simulink model "gm_flightController"  (R2018b)
settings: Solver=ode3  StartTime=0  StopTime=TFinal  FixedStep=Ts  RelTol=1e-3  EnableMultiTasking=on
libraries: hdlmdlgenlib x14
(part 1 of 2)
settings Model: Creator=The MathWorks, Inc.  LastModifiedBy=asus
settings SolverCC: MinimalZcImpactIntegration=on
settings DataIOCC: LimitDataPoints=on  SaveFormat=Array
settings OptimizationCC: BlockReduction=off  ConditionallyExecuteInputs=off  DefaultParameterBehavior=Inlined  BufferReuse=off  PassReuseOutputArgsThreshold=0
settings DebuggingCC: AlgebraicLoopMsg=none  InheritedTsInSrcMsg=none  ParameterPrecisionLossMsg=none  ParameterTunabilityLossMsg=error  UnconnectedInputMsg=none  UnconnectedOutputMsg=none  UnconnectedLineMsg=none  BusObjectLabelMismatch=error  LibraryContextMissingDiagnostic=none  SFUnexpectedBacktrackingDiag=warning  SFNoUnconditionalDefaultTransitionDiag=warning  SFExecutionAtInitializationDiag=none
settings HardwareCC: ProdBitPerPointer=32  ProdBitPerSizeT=32  ProdBitPerPtrDiffT=32  ProdLargestAtomicInteger=Long  ProdWordSize=32  ProdHWDeviceType=ARM Compatible->ARM 9
settings ModelReferenceCC: ModelReferenceNumInstancesAllowed=Single  PropagateSignalLabelsOutOfModel=off
settings SFSimCC: SimUseLocalCustomCode=off
settings RTWCC: Description=Generic Real-Time Target  GenerateReport=on  RTWUseLocalCustomCode=off  LaunchReport=on
settings CodeAppCC: ForceParamTrailComments=on  MaxIdLength=63  OperatorAnnotations=on  StateflowObjectComments=on  MATLABSourceComments=on
settings GRTTargetCC: TargetLangStandard=C89/C90 (ANSI)
settings ConfigComp: CovMetricSettings=dw  CovHtmlReporting=on  CovSaveCumulativeToWorkspaceVar=on  CovSaveSingleToWorkspaceVar=on  CovExternalEMLEnable=off  CovSFcnEnable=off

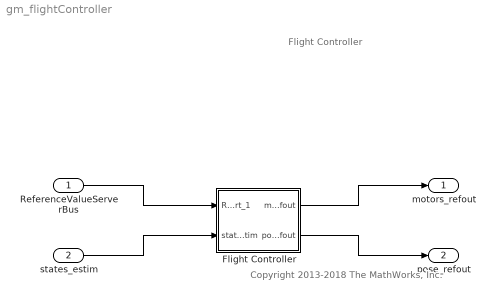
== system gm_flightController ==
  note: Copyright 2013-2018 The MathWorks, Inc.
  note: Flight Controller
  ReferenceValueServerBus : Inport  OutDataTypeStr=Bus: CommandBus  SampleTime=0.005  BusOutputAsStruct=on
  states_estim : Inport  Port=2  OutDataTypeStr=Bus: statesEstim_t  SampleTime=0.005  BusOutputAsStruct=on
  Flight Controller : Subsystem
  motors_refout : Outport
  pose_refout : Outport  Port=2
  wires:
  ReferenceValueServerBus/1 -> Flight Controller/1(ReferenceValueServerBus_Inport_1)
  states_estim/1 -> Flight Controller/2(states_estim)
  Flight Controller/1(motors_refout) -> motors_refout/1
  Flight Controller/2(pose_refout) -> pose_refout/1

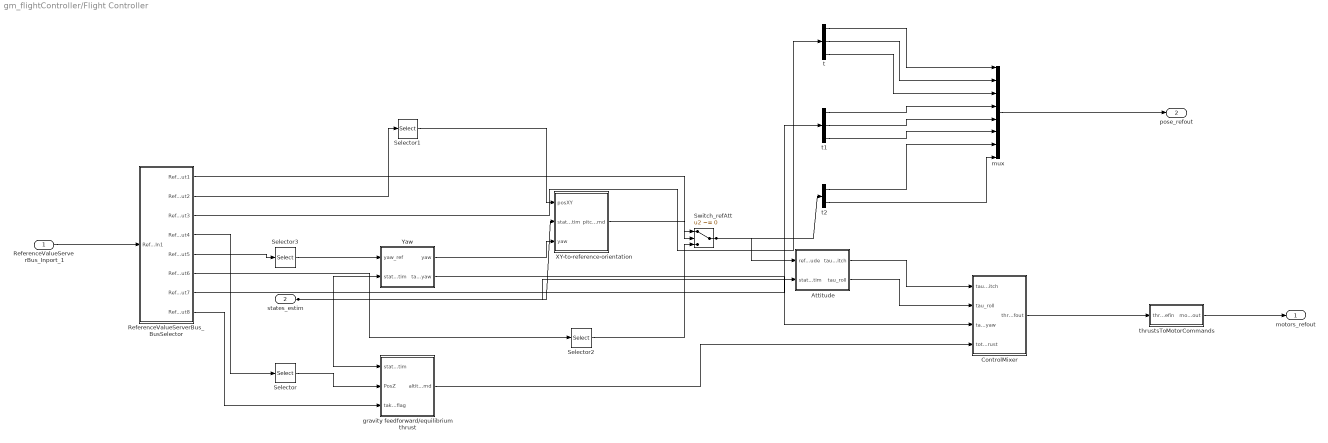
== system gm_flightController/Flight Controller ==
  ReferenceValueServerBus_Inport_1 : Inport  SampleTime=0.005
  states_estim : Inport  Port=2  SampleTime=0.005
  Attitude : Subsystem
  ControlMixer : Subsystem
  ReferenceValueServerBus_BusSelector : Subsystem
  Selector : Selector  SampleTime=0.005  IndexOptions=Index vector (dialog)  Indices=double(3)  OutputSizes=double(1)
  Selector1 : Selector  SampleTime=0.005  IndexOptions=Index vector (dialog)  Indices=double([1 2])  OutputSizes=double(1)
  Selector2 : Selector  SampleTime=0.005  IndexOptions=Index vector (dialog)  Indices=double([2 3])  OutputSizes=double(1)
  Selector3 : Selector  SampleTime=0.005  IndexOptions=Index vector (dialog)  Indices=double(1)  OutputSizes=double(1)
  Switch_refAtt : Switch  Criteria=u2 ~= 0  Threshold=double(0)  OutDataTypeStr=single  SampleTime=0.005
  XY-to-reference-orientation : Subsystem
  Yaw : Subsystem
  gravity feedforward/equilibrium thrust : Subsystem
  mux : Mux  Inputs=8
  t : Demux  Outputs=3
  t1 : Demux  Outputs=3
  t2 : Demux  Outputs=2
  thrustsToMotorCommands : Subsystem
  motors_refout : Outport
  pose_refout : Outport  Port=2
  wires:
  ReferenceValueServerBus_Inport_1/1 -> ReferenceValueServerBus_BusSelector/1(ReferenceValueServerBus_BusSelector_In1)
  states_estim/1 -> gravity feedforward/equilibrium thrust/1(states_estim), Attitude/2(states_estim), XY-to-reference-orientation/2(states_estim), Yaw/2(states_estim)
  Attitude/1(tau_pitch) -> ControlMixer/1(tau_pitch)
  Attitude/2(tau_roll) -> ControlMixer/2(tau_roll)
  ControlMixer/1(thrusts_refout) -> thrustsToMotorCommands/1(thrusts_refin)
  mux/1 -> pose_refout/1
  ReferenceValueServerBus_BusSelector/1(ReferenceValueServerBus_BusSelector_Out1) -> Switch_refAtt/2
  ReferenceValueServerBus_BusSelector/2(ReferenceValueServerBus_BusSelector_Out2) -> Selector1/1
  ReferenceValueServerBus_BusSelector/3(ReferenceValueServerBus_BusSelector_Out3) -> t/1
  ReferenceValueServerBus_BusSelector/4(ReferenceValueServerBus_BusSelector_Out4) -> Selector/1
  ReferenceValueServerBus_BusSelector/5(ReferenceValueServerBus_BusSelector_Out5) -> Selector3/1
  ReferenceValueServerBus_BusSelector/6(ReferenceValueServerBus_BusSelector_Out6) -> Selector2/1
  ReferenceValueServerBus_BusSelector/7(ReferenceValueServerBus_BusSelector_Out7) -> t1/1
  ReferenceValueServerBus_BusSelector/8(ReferenceValueServerBus_BusSelector_Out8) -> gravity feedforward/equilibrium thrust/3(takeoff_flag)
  Selector/1 -> gravity feedforward/equilibrium thrust/2(PosZ)
  Selector1/1 -> XY-to-reference-orientation/1(posXY)
  Selector2/1 -> Switch_refAtt/3
  Selector3/1 -> Yaw/1(yaw_ref)
  Switch_refAtt/1 -> t2/1, Attitude/1(refAttitude)
  XY-to-reference-orientation/1(pitch_roll_cmd) -> Switch_refAtt/1
  Yaw/1(yaw) -> XY-to-reference-orientation/3(yaw)
  Yaw/2(tau_yaw) -> ControlMixer/3(tau_yaw)
  gravity feedforward/equilibrium thrust/1(altitude_cmd) -> ControlMixer/4(totalThrust)
  thrustsToMotorCommands/1(motors_cmdout) -> motors_refout/1
  t/1 -> mux/1
  t/2 -> mux/2
  t/3 -> mux/3
  t1/1 -> mux/4
  t1/2 -> mux/5
  t1/3 -> mux/6
  t2/1 -> mux/7
  t2/2 -> mux/8

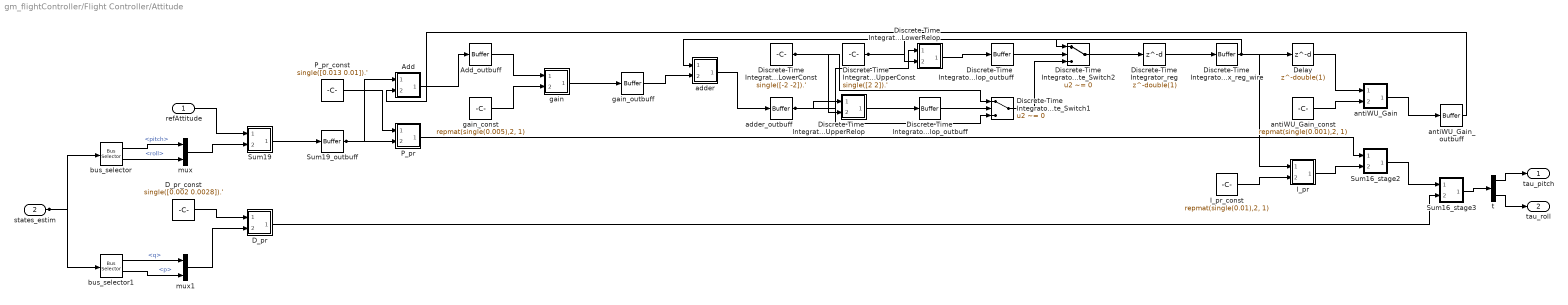
== system gm_flightController/Flight Controller/Attitude ==
  refAttitude : Inport  OutDataTypeStr=single  PortDimensions=[2]  SampleTime=0.005
  states_estim : Inport  Port=2  SampleTime=0.005
  Add : Subsystem
      mask Display: disp('NFP\nadd');
  Add_outbuff : hdlmdlgenlib/Buffer
      settings: SourceProductName=HDL Coder  SourceProductBaseCode=HD
  D_pr : Subsystem
      mask Display: disp('NFP\nmul');
  D_pr_const : Constant  Value=single([0.002 0.0028]).'  OutDataTypeStr=single  SampleTime=-1
  Delay : Delay  DelayLength=double(1)  InitialCondition=0  InputProcessing=Inherited  SampleTime=0.005
  Discrete-Time Integrator_reg : Delay  DelayLength=double(1)  InitialCondition=0  InputProcessing=Inherited  SampleTime=0.005
  Discrete-Time Integrator_saturate_LowerConst : Constant  Value=single([-2 -2]).'  OutDataTypeStr=single  SampleTime=-1
  Discrete-Time Integrator_saturate_LowerRelop : Subsystem
      mask Display: disp('NFP\nrelop');
  Discrete-Time Integrator_saturate_LowerRelop_outbuff : hdlmdlgenlib/Buffer
      settings: SourceProductName=HDL Coder  SourceProductBaseCode=HD
  Discrete-Time Integrator_saturate_Switch1 : Switch  Criteria=u2 ~= 0  Threshold=double(0)  OutDataTypeStr=single  SampleTime=0.005
  Discrete-Time Integrator_saturate_Switch2 : Switch  Criteria=u2 ~= 0  Threshold=double(0)  OutDataTypeStr=single  SampleTime=0.005
  Discrete-Time Integrator_saturate_UpperConst : Constant  Value=single([2 2]).'  OutDataTypeStr=single  SampleTime=-1
  Discrete-Time Integrator_saturate_UpperRelop : Subsystem
      mask Display: disp('NFP\nrelop');
  Discrete-Time Integrator_saturate_UpperRelop_outbuff : hdlmdlgenlib/Buffer
      settings: SourceProductName=HDL Coder  SourceProductBaseCode=HD
  Discrete-Time Integrator_x_reg_wire : hdlmdlgenlib/Buffer
      settings: SourceProductName=HDL Coder  SourceProductBaseCode=HD
  I_pr : Subsystem
      mask Display: disp('NFP\nmul');
  I_pr_const : Constant  Value=repmat(single(0.01),2, 1)  OutDataTypeStr=single  SampleTime=-1
  P_pr : Subsystem
      mask Display: disp('NFP\nmul');
  P_pr_const : Constant  Value=single([0.013 0.01]).'  OutDataTypeStr=single  SampleTime=-1
  Sum16_stage2 : Subsystem
      mask Display: disp('NFP\nadd');
  Sum16_stage3 : Subsystem
      mask Display: disp('NFP\nadd');
  Sum19 : Subsystem
      mask Display: disp('NFP\nadd');
  Sum19_outbuff : hdlmdlgenlib/Buffer
      settings: SourceProductName=HDL Coder  SourceProductBaseCode=HD
  adder : Subsystem
      mask Display: disp('NFP\nadd');
  adder_outbuff : hdlmdlgenlib/Buffer
      settings: SourceProductName=HDL Coder  SourceProductBaseCode=HD
  antiWU_Gain : Subsystem
      mask Display: disp('NFP\nmul');
  antiWU_Gain_const : Constant  Value=repmat(single(0.001),2, 1)  OutDataTypeStr=single  SampleTime=-1
  antiWU_Gain_outbuff : hdlmdlgenlib/Buffer
      settings: SourceProductName=HDL Coder  SourceProductBaseCode=HD
  bus_selector : BusSelector  OutputSignals=pitch,roll
  bus_selector1 : BusSelector  OutputSignals=q,p
  gain : Subsystem
      mask Display: disp('NFP\nmul');
  gain_const : Constant  Value=repmat(single(0.005),2, 1)  OutDataTypeStr=single  SampleTime=-1
  gain_outbuff : hdlmdlgenlib/Buffer
      settings: SourceProductName=HDL Coder  SourceProductBaseCode=HD
  mux : Mux  Inputs=2
  mux1 : Mux  Inputs=2
  t : Demux  Outputs=2
  tau_pitch : Outport
  tau_roll : Outport  Port=2
  wires:
  refAttitude/1 -> Sum19/1(In1)
  states_estim/1 -> bus_selector1/1, bus_selector/1
  Add_outbuff/1 -> gain/1(In1)
  bus_selector/1 -> mux/1  "<pitch>"
  bus_selector/2 -> mux/2  "<roll>"
  bus_selector1/1 -> mux1/1  "<q>"
  bus_selector1/2 -> mux1/2  "<p>"
  Delay/1 -> antiWU_Gain/1(In1)
  Discrete-Time Integrator_x_reg_wire/1 -> I_pr/1(In1), adder/1(In1), Delay/1
  mux/1 -> Sum19/2(In2)
  mux1/1 -> D_pr/2(In2)
  Sum19_outbuff/1 -> P_pr/2(In2), Add/1(In1)
  antiWU_Gain_outbuff/1 -> Add/2(In2)
  gain_outbuff/1 -> adder/2(In2)
  adder_outbuff/1 -> Discrete-Time Integrator_saturate_LowerRelop/1(In1), Discrete-Time Integrator_saturate_UpperRelop/1(In1), Discrete-Time Integrator_saturate_Switch1/3
  Discrete-Time Integrator_saturate_Switch2/1 -> Discrete-Time Integrator_reg/1
  Discrete-Time Integrator_saturate_LowerConst/1 -> Discrete-Time Integrator_saturate_UpperRelop/2(In2), Discrete-Time Integrator_saturate_Switch1/1
  Discrete-Time Integrator_saturate_UpperConst/1 -> Discrete-Time Integrator_saturate_LowerRelop/2(In2), Discrete-Time Integrator_saturate_Switch2/1
  Discrete-Time Integrator_saturate_UpperRelop_outbuff/1 -> Discrete-Time Integrator_saturate_Switch1/2
  Discrete-Time Integrator_saturate_LowerRelop_outbuff/1 -> Discrete-Time Integrator_saturate_Switch2/2
  Discrete-Time Integrator_saturate_Switch1/1 -> Discrete-Time Integrator_saturate_Switch2/3
  Discrete-Time Integrator_reg/1 -> Discrete-Time Integrator_x_reg_wire/1
  t/1 -> tau_pitch/1
  t/2 -> tau_roll/1
  D_pr_const/1 -> D_pr/1(In1)
  gain_const/1 -> gain/2(In2)
  I_pr_const/1 -> I_pr/2(In2)
  P_pr_const/1 -> P_pr/1(In1)
  antiWU_Gain_const/1 -> antiWU_Gain/2(In2)
  adder/1(Out1) -> adder_outbuff/1
  Discrete-Time Integrator_saturate_UpperRelop/1(Out1) -> Discrete-Time Integrator_saturate_UpperRelop_outbuff/1
  Discrete-Time Integrator_saturate_LowerRelop/1(Out1) -> Discrete-Time Integrator_saturate_LowerRelop_outbuff/1
  Add/1(Out1) -> Add_outbuff/1
  Sum16_stage2/1(Out1) -> Sum16_stage3/1(In1)
  Sum16_stage3/1(Out1) -> t/1
  Sum19/1(Out1) -> Sum19_outbuff/1
  D_pr/1(Out1) -> Sum16_stage3/2(In2)
  gain/1(Out1) -> gain_outbuff/1
  I_pr/1(Out1) -> Sum16_stage2/2(In2)
  P_pr/1(Out1) -> Sum16_stage2/1(In1)
  antiWU_Gain/1(Out1) -> antiWU_Gain_outbuff/1

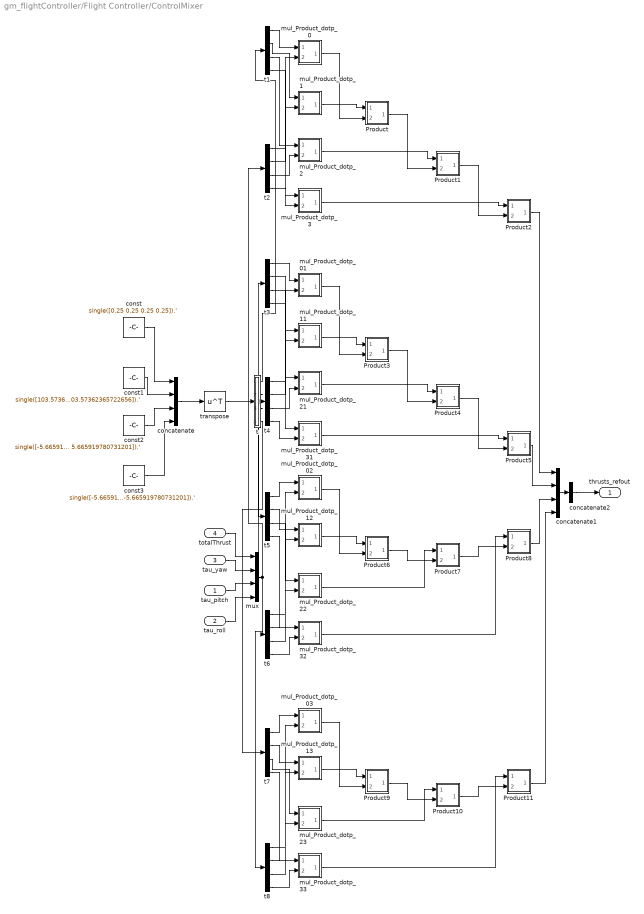
== system gm_flightController/Flight Controller/ControlMixer ==
  tau_pitch : Inport  OutDataTypeStr=single  PortDimensions=1  SampleTime=0.005
  tau_roll : Inport  Port=2  OutDataTypeStr=single  PortDimensions=1  SampleTime=0.005
  tau_yaw : Inport  Port=3  OutDataTypeStr=single  PortDimensions=1  SampleTime=0.005
  totalThrust : Inport  Port=4  OutDataTypeStr=single  PortDimensions=1  SampleTime=0.005
  Product : Subsystem
      mask Display: disp('NFP\nadd');
  Product1 : Subsystem
      mask Display: disp('NFP\nadd');
  Product10 : Subsystem
      mask Display: disp('NFP\nadd');
  Product11 : Subsystem
      mask Display: disp('NFP\nadd');
  Product2 : Subsystem
      mask Display: disp('NFP\nadd');
  Product3 : Subsystem
      mask Display: disp('NFP\nadd');
  Product4 : Subsystem
      mask Display: disp('NFP\nadd');
  Product5 : Subsystem
      mask Display: disp('NFP\nadd');
  Product6 : Subsystem
      mask Display: disp('NFP\nadd');
  Product7 : Subsystem
      mask Display: disp('NFP\nadd');
  Product8 : Subsystem
      mask Display: disp('NFP\nadd');
  Product9 : Subsystem
      mask Display: disp('NFP\nadd');
  concatenate : Concatenate  NumInputs=4  Mode=Multidimensional array  ConcatenateDimension=2
  concatenate1 : Concatenate  NumInputs=4
  concatenate2 : Concatenate  NumInputs=1  Mode=Multidimensional array  ConcatenateDimension=2
  const : Constant  Value=single([0.25 0.25 0.25 0.25]).'  OutDataTypeStr=single  SampleTime=-1
  const1 : Constant  Value=single([103.57362365722656 -103.57362365722656 103.57362365722656 -103.57362365722656]).'  OutDataTypeStr=single  SampleTime=-1
  const2 : Constant  Value=single([-5.665919780731201 -5.665919780731201 5.665919780731201 5.665919780731201]).'  OutDataTypeStr=single  SampleTime=-1
  const3 : Constant  Value=single([-5.665919780731201 5.665919780731201 5.665919780731201 -5.665919780731201]).'  OutDataTypeStr=single  SampleTime=-1
  mul_Product_dotp_0 : Subsystem
      mask Display: disp('NFP\nmul');
  mul_Product_dotp_01 : Subsystem
      mask Display: disp('NFP\nmul');
  mul_Product_dotp_02 : Subsystem
      mask Display: disp('NFP\nmul');
  mul_Product_dotp_03 : Subsystem
      mask Display: disp('NFP\nmul');
  mul_Product_dotp_1 : Subsystem
      mask Display: disp('NFP\nmul');
  mul_Product_dotp_11 : Subsystem
      mask Display: disp('NFP\nmul');
  mul_Product_dotp_12 : Subsystem
      mask Display: disp('NFP\nmul');
  mul_Product_dotp_13 : Subsystem
      mask Display: disp('NFP\nmul');
  mul_Product_dotp_2 : Subsystem
      mask Display: disp('NFP\nmul');
  mul_Product_dotp_21 : Subsystem
      mask Display: disp('NFP\nmul');
  mul_Product_dotp_22 : Subsystem
      mask Display: disp('NFP\nmul');
  mul_Product_dotp_23 : Subsystem
      mask Display: disp('NFP\nmul');
  mul_Product_dotp_3 : Subsystem
      mask Display: disp('NFP\nmul');
  mul_Product_dotp_31 : Subsystem
      mask Display: disp('NFP\nmul');
  mul_Product_dotp_32 : Subsystem
      mask Display: disp('NFP\nmul');
  mul_Product_dotp_33 : Subsystem
      mask Display: disp('NFP\nmul');
  mux : Mux
  t : Subsystem
  t{1..8} (8 alike) : Demux
  transpose : Math  Operator=transpose  SaturateOnIntegerOverflow=on
  thrusts_refout : Outport
  wires:
  tau_pitch/1 -> mux/3
  tau_roll/1 -> mux/4
  tau_yaw/1 -> mux/2
  totalThrust/1 -> mux/1
  mux/1 -> t8/1, t6/1, t4/1, t2/1
  concatenate2/1 -> thrusts_refout/1
  concatenate/1 -> transpose/1
  const/1 -> concatenate/1
  const1/1 -> concatenate/2
  const2/1 -> concatenate/3
  const3/1 -> concatenate/4
  transpose/1 -> t/1(in0)
  t/1(out0) -> t1/1
  t/2(out1) -> t3/1
  t/3(out2) -> t5/1
  t/4(out3) -> t7/1
  t1/1 -> mul_Product_dotp_0/1(In1)
  t1/2 -> mul_Product_dotp_1/1(In1)
  t1/3 -> mul_Product_dotp_2/1(In1)
  t1/4 -> mul_Product_dotp_3/1(In1)
  t2/1 -> mul_Product_dotp_0/2(In2)
  t2/2 -> mul_Product_dotp_1/2(In2)
  t2/3 -> mul_Product_dotp_2/2(In2)
  t2/4 -> mul_Product_dotp_3/2(In2)
  t3/1 -> mul_Product_dotp_01/1(In1)
  t3/2 -> mul_Product_dotp_11/1(In1)
  t3/3 -> mul_Product_dotp_21/1(In1)
  t3/4 -> mul_Product_dotp_31/1(In1)
  t4/1 -> mul_Product_dotp_01/2(In2)
  t4/2 -> mul_Product_dotp_11/2(In2)
  t4/3 -> mul_Product_dotp_21/2(In2)
  t4/4 -> mul_Product_dotp_31/2(In2)
  t5/1 -> mul_Product_dotp_02/1(In1)
  t5/2 -> mul_Product_dotp_12/1(In1)
  t5/3 -> mul_Product_dotp_22/1(In1)
  t5/4 -> mul_Product_dotp_32/1(In1)
  t6/1 -> mul_Product_dotp_02/2(In2)
  t6/2 -> mul_Product_dotp_12/2(In2)
  t6/3 -> mul_Product_dotp_22/2(In2)
  t6/4 -> mul_Product_dotp_32/2(In2)
  t7/1 -> mul_Product_dotp_03/1(In1)
  t7/2 -> mul_Product_dotp_13/1(In1)
  t7/3 -> mul_Product_dotp_23/1(In1)
  t7/4 -> mul_Product_dotp_33/1(In1)
  t8/1 -> mul_Product_dotp_03/2(In2)
  t8/2 -> mul_Product_dotp_13/2(In2)
  t8/3 -> mul_Product_dotp_23/2(In2)
  t8/4 -> mul_Product_dotp_33/2(In2)
  concatenate1/1 -> concatenate2/1
  mul_Product_dotp_0/1(Out1) -> Product/2(In2)
  mul_Product_dotp_1/1(Out1) -> Product/1(In1)
  Product/1(Out1) -> Product1/2(In2)
  mul_Product_dotp_2/1(Out1) -> Product1/1(In1)
  Product1/1(Out1) -> Product2/2(In2)
  mul_Product_dotp_3/1(Out1) -> Product2/1(In1)
  Product2/1(Out1) -> concatenate1/1
  mul_Product_dotp_01/1(Out1) -> Product3/2(In2)
  mul_Product_dotp_11/1(Out1) -> Product3/1(In1)
  Product3/1(Out1) -> Product4/2(In2)
  mul_Product_dotp_21/1(Out1) -> Product4/1(In1)
  Product4/1(Out1) -> Product5/2(In2)
  mul_Product_dotp_31/1(Out1) -> Product5/1(In1)
  Product5/1(Out1) -> concatenate1/2
  mul_Product_dotp_02/1(Out1) -> Product6/2(In2)
  mul_Product_dotp_12/1(Out1) -> Product6/1(In1)
  Product6/1(Out1) -> Product7/2(In2)
  mul_Product_dotp_22/1(Out1) -> Product7/1(In1)
  Product7/1(Out1) -> Product8/2(In2)
  mul_Product_dotp_32/1(Out1) -> Product8/1(In1)
  Product8/1(Out1) -> concatenate1/3
  mul_Product_dotp_03/1(Out1) -> Product9/2(In2)
  mul_Product_dotp_13/1(Out1) -> Product9/1(In1)
  Product9/1(Out1) -> Product10/2(In2)
  mul_Product_dotp_23/1(Out1) -> Product10/1(In1)
  Product10/1(Out1) -> Product11/2(In2)
  mul_Product_dotp_33/1(Out1) -> Product11/1(In1)
  Product11/1(Out1) -> concatenate1/4

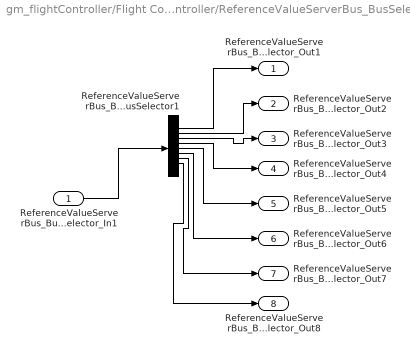
== system gm_flightController/Flight Controller/ReferenceValueServerBus_BusSelector ==
  ReferenceValueServerBus_BusSelector_In1 : Inport  SampleTime=0.005
  ReferenceValueServerBus_BusSelector_BusSelector1 : BusSelector  DisableCoverage=on  OutputSignals=controlModePosVSOrient,pos_ref,pos_ref,pos_ref,orient_ref,orient_ref,orient_ref,takeoff_flag
  ReferenceValueServerBus_BusSelector_Out1 : Outport
  ReferenceValueServerBus_BusSelector_Out2 : Outport  Port=2
  ReferenceValueServerBus_BusSelector_Out3 : Outport  Port=3
  ReferenceValueServerBus_BusSelector_Out4 : Outport  Port=4
  ReferenceValueServerBus_BusSelector_Out5 : Outport  Port=5
  ReferenceValueServerBus_BusSelector_Out6 : Outport  Port=6
  ReferenceValueServerBus_BusSelector_Out7 : Outport  Port=7
  ReferenceValueServerBus_BusSelector_Out8 : Outport  Port=8
  wires:
  ReferenceValueServerBus_BusSelector_In1/1 -> ReferenceValueServerBus_BusSelector_BusSelector1/1
  ReferenceValueServerBus_BusSelector_BusSelector1/1 -> ReferenceValueServerBus_BusSelector_Out1/1
  ReferenceValueServerBus_BusSelector_BusSelector1/2 -> ReferenceValueServerBus_BusSelector_Out2/1
  ReferenceValueServerBus_BusSelector_BusSelector1/3 -> ReferenceValueServerBus_BusSelector_Out3/1
  ReferenceValueServerBus_BusSelector_BusSelector1/4 -> ReferenceValueServerBus_BusSelector_Out4/1
  ReferenceValueServerBus_BusSelector_BusSelector1/5 -> ReferenceValueServerBus_BusSelector_Out5/1
  ReferenceValueServerBus_BusSelector_BusSelector1/6 -> ReferenceValueServerBus_BusSelector_Out6/1
  ReferenceValueServerBus_BusSelector_BusSelector1/7 -> ReferenceValueServerBus_BusSelector_Out7/1
  ReferenceValueServerBus_BusSelector_BusSelector1/8 -> ReferenceValueServerBus_BusSelector_Out8/1

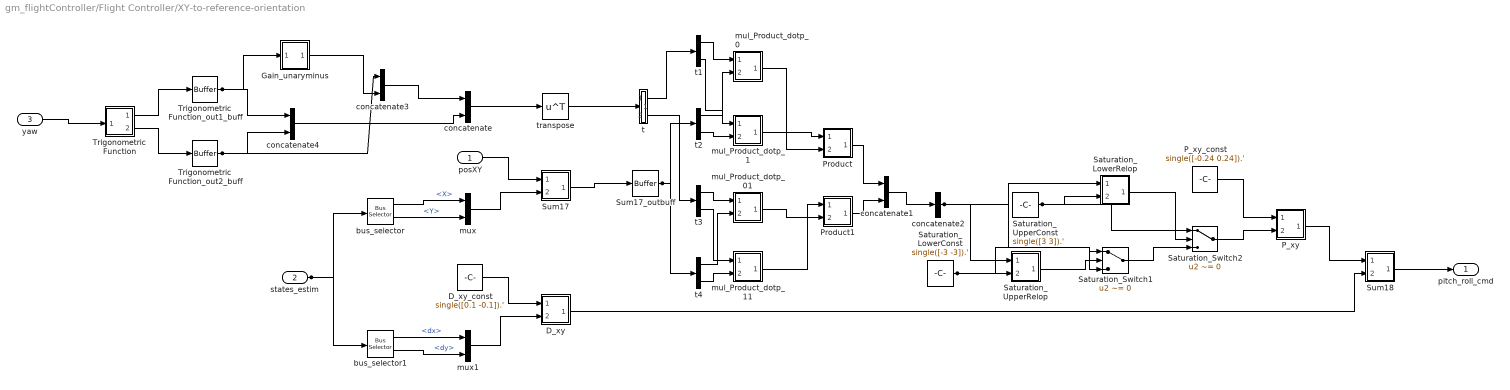
== system gm_flightController/Flight Controller/XY-to-reference-orientation ==
  posXY : Inport  OutDataTypeStr=single  PortDimensions=[2]  SampleTime=0.005
  states_estim : Inport  Port=2  SampleTime=0.005
  yaw : Inport  Port=3  OutDataTypeStr=single  PortDimensions=1  SampleTime=0.005
  D_xy : Subsystem
      mask Display: disp('NFP\nmul');
  D_xy_const : Constant  Value=single([0.1 -0.1]).'  OutDataTypeStr=single  SampleTime=-1
  Gain_unaryminus : Subsystem
      mask Display: disp('NFP\numinus');
  P_xy : Subsystem
      mask Display: disp('NFP\nmul');
  P_xy_const : Constant  Value=single([-0.24 0.24]).'  OutDataTypeStr=single  SampleTime=-1
  Product : Subsystem
      mask Display: disp('NFP\nadd');
  Product1 : Subsystem
      mask Display: disp('NFP\nadd');
  Saturation_LowerConst : Constant  Value=single([-3 -3]).'  OutDataTypeStr=single  SampleTime=-1
  Saturation_LowerRelop : Subsystem
      mask Display: disp('NFP\nrelop');
  Saturation_Switch1 : Switch  Criteria=u2 ~= 0  Threshold=double(0)  OutDataTypeStr=single  SampleTime=0.005
  Saturation_Switch2 : Switch  Criteria=u2 ~= 0  Threshold=double(0)  OutDataTypeStr=single  SampleTime=0.005
  Saturation_UpperConst : Constant  Value=single([3 3]).'  OutDataTypeStr=single  SampleTime=-1
  Saturation_UpperRelop : Subsystem
      mask Display: disp('NFP\nrelop');
  Sum17 : Subsystem
      mask Display: disp('NFP\nadd');
  Sum17_outbuff : hdlmdlgenlib/Buffer
      settings: SourceProductName=HDL Coder  SourceProductBaseCode=HD
  Sum18 : Subsystem
      mask Display: disp('NFP\nadd');
  Trigonometric Function : Subsystem
      mask Display: disp('NFP\ntrig2');
  Trigonometric Function_out1_buff : hdlmdlgenlib/Buffer
      settings: SourceProductName=HDL Coder  SourceProductBaseCode=HD
  Trigonometric Function_out2_buff : hdlmdlgenlib/Buffer
      settings: SourceProductName=HDL Coder  SourceProductBaseCode=HD
  bus_selector : BusSelector  OutputSignals=X,Y
  bus_selector1 : BusSelector  OutputSignals=dx,dy
  concatenate : Concatenate  Mode=Multidimensional array  ConcatenateDimension=2
  concatenate1 : Concatenate
  concatenate2 : Concatenate  NumInputs=1  Mode=Multidimensional array  ConcatenateDimension=2
  concatenate3 : Concatenate
  concatenate4 : Concatenate
  mul_Product_dotp_0 : Subsystem
      mask Display: disp('NFP\nmul');
  mul_Product_dotp_01 : Subsystem
      mask Display: disp('NFP\nmul');
  mul_Product_dotp_1 : Subsystem
      mask Display: disp('NFP\nmul');
  mul_Product_dotp_11 : Subsystem
      mask Display: disp('NFP\nmul');
  mux : Mux  Inputs=2
  mux1 : Mux  Inputs=2
  t : Subsystem
  t{1..4} (4 alike) : Demux  Outputs=2
  transpose : Math  Operator=transpose  SaturateOnIntegerOverflow=on
  pitch_roll_cmd : Outport
  wires:
  posXY/1 -> Sum17/1(In1)
  states_estim/1 -> bus_selector1/1, bus_selector/1
  yaw/1 -> Trigonometric Function/1(In1)
  bus_selector/1 -> mux/1  "<X>"
  bus_selector/2 -> mux/2  "<Y>"
  bus_selector1/1 -> mux1/1  "<dx>"
  bus_selector1/2 -> mux1/2  "<dy>"
  concatenate/1 -> transpose/1
  mux/1 -> Sum17/2(In2)
  mux1/1 -> D_xy/2(In2)
  concatenate2/1 -> Saturation_LowerRelop/1(In1), Saturation_UpperRelop/1(In1), Saturation_Switch1/3
  Saturation_Switch2/1 -> P_xy/2(In2)
  Sum17_outbuff/1 -> t4/1, t2/1
  Trigonometric Function_out1_buff/1 -> Gain_unaryminus/1(In1), concatenate4/1
  Trigonometric Function_out2_buff/1 -> concatenate4/2, concatenate3/1
  concatenate3/1 -> concatenate/1
  concatenate4/1 -> concatenate/2
  transpose/1 -> t/1(in0)
  t/1(out0) -> t1/1
  t/2(out1) -> t3/1
  t1/1 -> mul_Product_dotp_0/1(In1)
  t1/2 -> mul_Product_dotp_1/1(In1)
  t2/1 -> mul_Product_dotp_0/2(In2)
  t2/2 -> mul_Product_dotp_1/2(In2)
  t3/1 -> mul_Product_dotp_01/1(In1)
  t3/2 -> mul_Product_dotp_11/1(In1)
  t4/1 -> mul_Product_dotp_01/2(In2)
  t4/2 -> mul_Product_dotp_11/2(In2)
  concatenate1/1 -> concatenate2/1
  Saturation_LowerConst/1 -> Saturation_UpperRelop/2(In2), Saturation_Switch1/1
  Saturation_UpperConst/1 -> Saturation_LowerRelop/2(In2), Saturation_Switch2/1
  Saturation_Switch1/1 -> Saturation_Switch2/3
  D_xy_const/1 -> D_xy/1(In1)
  P_xy_const/1 -> P_xy/1(In1)
  Gain_unaryminus/1(Out1) -> concatenate3/2
  mul_Product_dotp_0/1(Out1) -> Product/2(In2)
  mul_Product_dotp_1/1(Out1) -> Product/1(In1)
  Product/1(Out1) -> concatenate1/1
  mul_Product_dotp_01/1(Out1) -> Product1/2(In2)
  mul_Product_dotp_11/1(Out1) -> Product1/1(In1)
  Product1/1(Out1) -> concatenate1/2
  Saturation_UpperRelop/1(Out1) -> Saturation_Switch1/2
  Saturation_LowerRelop/1(Out1) -> Saturation_Switch2/2
  Sum17/1(Out1) -> Sum17_outbuff/1
  Sum18/1(Out1) -> pitch_roll_cmd/1
  Trigonometric Function/1(Out1) -> Trigonometric Function_out1_buff/1
  Trigonometric Function/2(Out2) -> Trigonometric Function_out2_buff/1
  D_xy/1(Out1) -> Sum18/2(In2)
  P_xy/1(Out1) -> Sum18/1(In1)

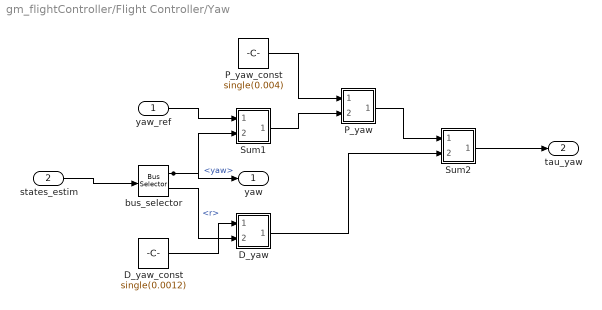
== system gm_flightController/Flight Controller/Yaw ==
  yaw_ref : Inport  OutDataTypeStr=single  PortDimensions=1  SampleTime=0.005
  states_estim : Inport  Port=2  SampleTime=0.005
  D_yaw : Subsystem
      mask Display: disp('NFP\nmul');
  D_yaw_const : Constant  Value=single(0.0012)  OutDataTypeStr=single  SampleTime=-1
  P_yaw : Subsystem
      mask Display: disp('NFP\nmul');
  P_yaw_const : Constant  Value=single(0.004)  OutDataTypeStr=single  SampleTime=-1
  Sum1 : Subsystem
      mask Display: disp('NFP\nadd');
  Sum2 : Subsystem
      mask Display: disp('NFP\nadd');
  bus_selector : BusSelector  OutputSignals=yaw,r
  yaw : Outport
  tau_yaw : Outport  Port=2
  wires:
  yaw_ref/1 -> Sum1/1(In1)
  states_estim/1 -> bus_selector/1
  bus_selector/1 -> Sum1/2(In2), yaw/1  "<yaw>"
  bus_selector/2 -> D_yaw/2(In2)  "<r>"
  D_yaw_const/1 -> D_yaw/1(In1)
  P_yaw_const/1 -> P_yaw/1(In1)
  Sum1/1(Out1) -> P_yaw/2(In2)
  Sum2/1(Out1) -> tau_yaw/1
  D_yaw/1(Out1) -> Sum2/2(In2)
  P_yaw/1(Out1) -> Sum2/1(In1)

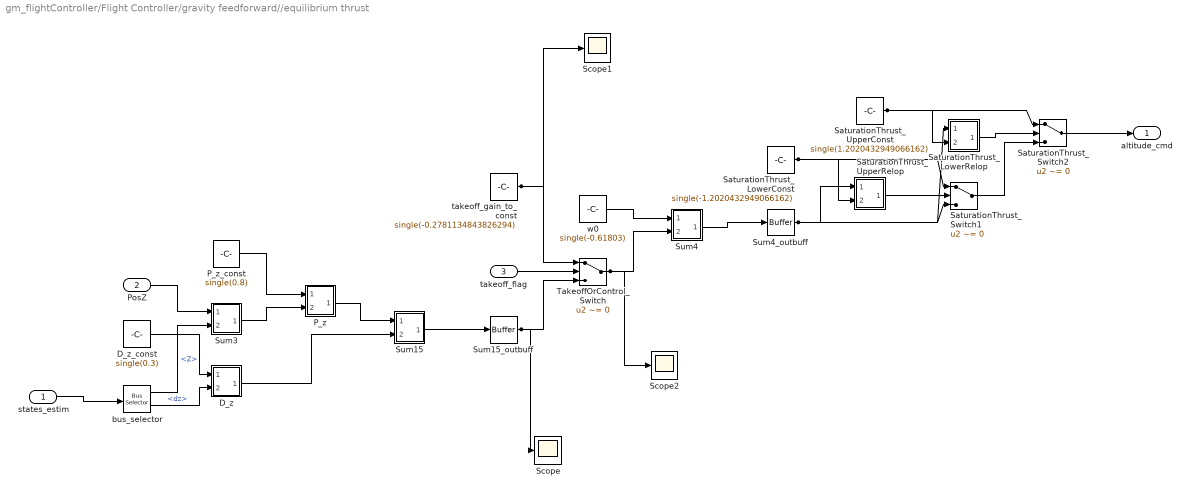
== system gm_flightController/Flight Controller/gravity feedforward//equilibrium thrust ==
  states_estim : Inport  SampleTime=0.005
  PosZ : Inport  Port=2  OutDataTypeStr=single  PortDimensions=1  SampleTime=0.005
  takeoff_flag : Inport  Port=3  OutDataTypeStr=boolean  PortDimensions=1  SampleTime=0.005
  D_z : Subsystem
      mask Display: disp('NFP\nmul');
  D_z_const : Constant  Value=single(0.3)  OutDataTypeStr=single  SampleTime=-1
  P_z : Subsystem
      mask Display: disp('NFP\nmul');
  P_z_const : Constant  Value=single(0.8)  OutDataTypeStr=single  SampleTime=-1
  SaturationThrust_LowerConst : Constant  Value=single(-1.2020432949066162)  OutDataTypeStr=single  SampleTime=-1
  SaturationThrust_LowerRelop : Subsystem
      mask Display: disp('NFP\nrelop');
  SaturationThrust_Switch1 : Switch  Criteria=u2 ~= 0  Threshold=double(0)  OutDataTypeStr=single  SampleTime=0.005
  SaturationThrust_Switch2 : Switch  Criteria=u2 ~= 0  Threshold=double(0)  OutDataTypeStr=single  SampleTime=0.005
  SaturationThrust_UpperConst : Constant  Value=single(1.2020432949066162)  OutDataTypeStr=single  SampleTime=-1
  SaturationThrust_UpperRelop : Subsystem
      mask Display: disp('NFP\nrelop');
  Scope : Scope
  Scope1 : Scope
  Scope2 : Scope
  Sum15 : Subsystem
      mask Display: disp('NFP\nadd');
  Sum15_outbuff : hdlmdlgenlib/Buffer
      settings: SourceProductName=HDL Coder  SourceProductBaseCode=HD
  Sum3 : Subsystem
      mask Display: disp('NFP\nadd');
  Sum4 : Subsystem
      mask Display: disp('NFP\nadd');
  Sum4_outbuff : hdlmdlgenlib/Buffer
      settings: SourceProductName=HDL Coder  SourceProductBaseCode=HD
  TakeoffOrControl_Switch : Switch  Criteria=u2 ~= 0  Threshold=double(0)  OutDataTypeStr=single  SampleTime=0.005
  bus_selector : BusSelector  OutputSignals=Z,dz
  takeoff_gain_to_const : Constant  Value=single(-0.2781134843826294)  OutDataTypeStr=single  SampleTime=-1
  w0 : Constant  Value=single(-0.61803)  OutDataTypeStr=single  SampleTime=-1
  altitude_cmd : Outport
  wires:
  states_estim/1 -> bus_selector/1
  PosZ/1 -> Sum3/1(In1)
  takeoff_flag/1 -> TakeoffOrControl_Switch/2
  bus_selector/1 -> Sum3/2(In2)  "<Z>"
  bus_selector/2 -> D_z/2(In2)  "<dz>"
  SaturationThrust_Switch2/1 -> altitude_cmd/1
  Sum15_outbuff/1 -> TakeoffOrControl_Switch/3, Scope/1
  Sum4_outbuff/1 -> SaturationThrust_LowerRelop/1(In1), SaturationThrust_UpperRelop/1(In1), SaturationThrust_Switch1/3
  TakeoffOrControl_Switch/1 -> Sum4/2(In2), Scope2/1
  takeoff_gain_to_const/1 -> TakeoffOrControl_Switch/1, Scope1/1
  w0/1 -> Sum4/1(In1)
  SaturationThrust_LowerConst/1 -> SaturationThrust_UpperRelop/2(In2), SaturationThrust_Switch1/1
  SaturationThrust_UpperConst/1 -> SaturationThrust_LowerRelop/2(In2), SaturationThrust_Switch2/1
  SaturationThrust_Switch1/1 -> SaturationThrust_Switch2/3
  D_z_const/1 -> D_z/1(In1)
  P_z_const/1 -> P_z/1(In1)
  SaturationThrust_UpperRelop/1(Out1) -> SaturationThrust_Switch1/2
  SaturationThrust_LowerRelop/1(Out1) -> SaturationThrust_Switch2/2
  Sum15/1(Out1) -> Sum15_outbuff/1
  Sum3/1(Out1) -> P_z/2(In2)
  Sum4/1(Out1) -> Sum4_outbuff/1
  D_z/1(Out1) -> Sum15/2(In2)
  P_z/1(Out1) -> Sum15/1(In1)

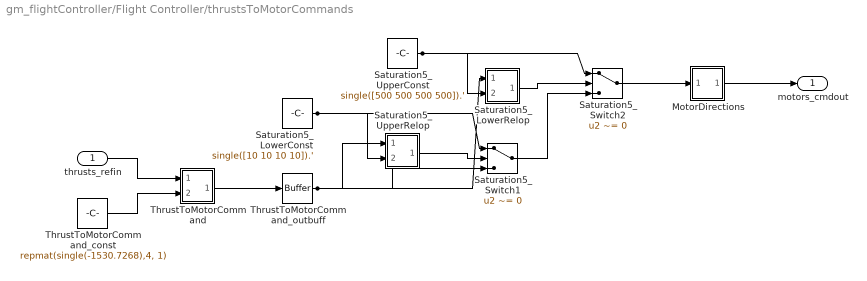
== system gm_flightController/Flight Controller/thrustsToMotorCommands ==
  thrusts_refin : Inport  OutDataTypeStr=single  PortDimensions=[4]  SampleTime=0.005
  MotorDirections : Subsystem
      mask Display: disp('NFP\ngain_pow2');
  Saturation5_LowerConst : Constant  Value=single([10 10 10 10]).'  OutDataTypeStr=single  SampleTime=-1
  Saturation5_LowerRelop : Subsystem
      mask Display: disp('NFP\nrelop');
  Saturation5_Switch1 : Switch  Criteria=u2 ~= 0  Threshold=double(0)  OutDataTypeStr=single  SampleTime=0.005
  Saturation5_Switch2 : Switch  Criteria=u2 ~= 0  Threshold=double(0)  OutDataTypeStr=single  SampleTime=0.005
  Saturation5_UpperConst : Constant  Value=single([500 500 500 500]).'  OutDataTypeStr=single  SampleTime=-1
  Saturation5_UpperRelop : Subsystem
      mask Display: disp('NFP\nrelop');
  ThrustToMotorCommand : Subsystem
      mask Display: disp('NFP\nmul');
  ThrustToMotorCommand_const : Constant  Value=repmat(single(-1530.7268),4, 1)  OutDataTypeStr=single  SampleTime=-1
  ThrustToMotorCommand_outbuff : hdlmdlgenlib/Buffer
      settings: SourceProductName=HDL Coder  SourceProductBaseCode=HD
  motors_cmdout : Outport
  wires:
  thrusts_refin/1 -> ThrustToMotorCommand/1(In1)
  Saturation5_Switch2/1 -> MotorDirections/1(In1)
  ThrustToMotorCommand_outbuff/1 -> Saturation5_LowerRelop/1(In1), Saturation5_UpperRelop/1(In1), Saturation5_Switch1/3
  Saturation5_LowerConst/1 -> Saturation5_UpperRelop/2(In2), Saturation5_Switch1/1
  Saturation5_UpperConst/1 -> Saturation5_LowerRelop/2(In2), Saturation5_Switch2/1
  Saturation5_Switch1/1 -> Saturation5_Switch2/3
  ThrustToMotorCommand_const/1 -> ThrustToMotorCommand/2(In2)
  MotorDirections/1(Out1) -> motors_cmdout/1
  Saturation5_UpperRelop/1(Out1) -> Saturation5_Switch1/2
  Saturation5_LowerRelop/1(Out1) -> Saturation5_Switch2/2
  ThrustToMotorCommand/1(Out1) -> ThrustToMotorCommand_outbuff/1

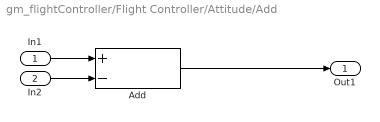
== system gm_flightController/Flight Controller/Attitude/Add ==
  In1 : Inport
  In2 : Inport  Port=2
  Add : Sum  Inputs=+-  OutDataTypeStr=single  SampleTime=0.005  SaturateOnIntegerOverflow=on  InputSameDT=on
  Out1 : Outport
  wires:
  In1/1 -> Add/1
  In2/1 -> Add/2
  Add/1 -> Out1/1

== system gm_flightController/Flight Controller/Attitude/D_pr ==
  In1 : Inport
  In2 : Inport  Port=2
  D_pr : Product  Inputs=**  OutDataTypeStr=single  SampleTime=0.005
  Out1 : Outport
  wires:
  In1/1 -> D_pr/1
  In2/1 -> D_pr/2
  D_pr/1 -> Out1/1

== system gm_flightController/Flight Controller/Attitude/Discrete-Time Integrator_saturate_LowerRelop ==
  In1 : Inport
  In2 : Inport  Port=2
  Discrete-Time Integrator_saturate_LowerRelop : RelationalOperator  Operator=>  OutDataTypeStr=boolean  SampleTime=0.005  RndMeth=Nearest
  Out1 : Outport
  wires:
  In1/1 -> Discrete-Time Integrator_saturate_LowerRelop/1
  In2/1 -> Discrete-Time Integrator_saturate_LowerRelop/2
  Discrete-Time Integrator_saturate_LowerRelop/1 -> Out1/1

== system gm_flightController/Flight Controller/Attitude/Discrete-Time Integrator_saturate_UpperRelop ==
  In1 : Inport
  In2 : Inport  Port=2
  Discrete-Time Integrator_saturate_UpperRelop : RelationalOperator  Operator=<  OutDataTypeStr=boolean  SampleTime=0.005  RndMeth=Nearest
  Out1 : Outport
  wires:
  In1/1 -> Discrete-Time Integrator_saturate_UpperRelop/1
  In2/1 -> Discrete-Time Integrator_saturate_UpperRelop/2
  Discrete-Time Integrator_saturate_UpperRelop/1 -> Out1/1

== system gm_flightController/Flight Controller/Attitude/I_pr ==
  In1 : Inport
  In2 : Inport  Port=2
  I_pr : Product  Inputs=**  OutDataTypeStr=single  SampleTime=0.005
  Out1 : Outport
  wires:
  In1/1 -> I_pr/1
  In2/1 -> I_pr/2
  I_pr/1 -> Out1/1

== system gm_flightController/Flight Controller/Attitude/P_pr ==
  In1 : Inport
  In2 : Inport  Port=2
  P_pr : Product  Inputs=**  OutDataTypeStr=single  SampleTime=0.005
  Out1 : Outport
  wires:
  In1/1 -> P_pr/1
  In2/1 -> P_pr/2
  P_pr/1 -> Out1/1

== system gm_flightController/Flight Controller/Attitude/Sum16_stage2 ==
  In1 : Inport
  In2 : Inport  Port=2
  Sum16_stage2 : Sum  OutDataTypeStr=single  SampleTime=0.005  SaturateOnIntegerOverflow=on  InputSameDT=on
  Out1 : Outport
  wires:
  In1/1 -> Sum16_stage2/1
  In2/1 -> Sum16_stage2/2
  Sum16_stage2/1 -> Out1/1

== system gm_flightController/Flight Controller/Attitude/Sum16_stage3 ==
  In1 : Inport
  In2 : Inport  Port=2
  Sum16_stage3 : Sum  Inputs=+-  OutDataTypeStr=single  SampleTime=0.005  SaturateOnIntegerOverflow=on  InputSameDT=on
  Out1 : Outport
  wires:
  In1/1 -> Sum16_stage3/1
  In2/1 -> Sum16_stage3/2
  Sum16_stage3/1 -> Out1/1

== system gm_flightController/Flight Controller/Attitude/Sum19 ==
  In1 : Inport
  In2 : Inport  Port=2
  Sum19 : Sum  Inputs=+-  OutDataTypeStr=single  SampleTime=0.005  SaturateOnIntegerOverflow=on  InputSameDT=on
  Out1 : Outport
  wires:
  In1/1 -> Sum19/1
  In2/1 -> Sum19/2
  Sum19/1 -> Out1/1

== system gm_flightController/Flight Controller/Attitude/adder ==
  In1 : Inport
  In2 : Inport  Port=2
  adder : Sum  OutDataTypeStr=single  SampleTime=0.005  SaturateOnIntegerOverflow=on  InputSameDT=on
  Out1 : Outport
  wires:
  In1/1 -> adder/1
  In2/1 -> adder/2
  adder/1 -> Out1/1

== system gm_flightController/Flight Controller/Attitude/antiWU_Gain ==
  In1 : Inport
  In2 : Inport  Port=2
  antiWU_Gain : Product  Inputs=**  OutDataTypeStr=single  SampleTime=0.005
  Out1 : Outport
  wires:
  In1/1 -> antiWU_Gain/1
  In2/1 -> antiWU_Gain/2
  antiWU_Gain/1 -> Out1/1

== system gm_flightController/Flight Controller/Attitude/gain ==
  In1 : Inport
  In2 : Inport  Port=2
  gain : Product  Inputs=**  OutDataTypeStr=single  SampleTime=0.005
  Out1 : Outport
  wires:
  In1/1 -> gain/1
  In2/1 -> gain/2
  gain/1 -> Out1/1

== system gm_flightController/Flight Controller/ControlMixer/Product ==
  In1 : Inport
  In2 : Inport  Port=2
  Product : Sum  OutDataTypeStr=single  RndMeth=Zero  SampleTime=0.005  SaturateOnIntegerOverflow=on  InputSameDT=on
  Out1 : Outport
  wires:
  In1/1 -> Product/1
  In2/1 -> Product/2
  Product/1 -> Out1/1

== system gm_flightController/Flight Controller/ControlMixer/Product1 ==
  In1 : Inport
  In2 : Inport  Port=2
  Product1 : Sum  OutDataTypeStr=single  RndMeth=Zero  SampleTime=0.005  SaturateOnIntegerOverflow=on  InputSameDT=on
  Out1 : Outport
  wires:
  In1/1 -> Product1/1
  In2/1 -> Product1/2
  Product1/1 -> Out1/1

== system gm_flightController/Flight Controller/ControlMixer/Product10 ==
  In1 : Inport
  In2 : Inport  Port=2
  Product10 : Sum  OutDataTypeStr=single  RndMeth=Zero  SampleTime=0.005  SaturateOnIntegerOverflow=on  InputSameDT=on
  Out1 : Outport
  wires:
  In1/1 -> Product10/1
  In2/1 -> Product10/2
  Product10/1 -> Out1/1

== system gm_flightController/Flight Controller/ControlMixer/Product11 ==
  In1 : Inport
  In2 : Inport  Port=2
  Product11 : Sum  OutDataTypeStr=single  RndMeth=Zero  SampleTime=0.005  SaturateOnIntegerOverflow=on  InputSameDT=on
  Out1 : Outport
  wires:
  In1/1 -> Product11/1
  In2/1 -> Product11/2
  Product11/1 -> Out1/1

== system gm_flightController/Flight Controller/ControlMixer/Product2 ==
  In1 : Inport
  In2 : Inport  Port=2
  Product2 : Sum  OutDataTypeStr=single  RndMeth=Zero  SampleTime=0.005  SaturateOnIntegerOverflow=on  InputSameDT=on
  Out1 : Outport
  wires:
  In1/1 -> Product2/1
  In2/1 -> Product2/2
  Product2/1 -> Out1/1

== system gm_flightController/Flight Controller/ControlMixer/Product3 ==
  In1 : Inport
  In2 : Inport  Port=2
  Product3 : Sum  OutDataTypeStr=single  RndMeth=Zero  SampleTime=0.005  SaturateOnIntegerOverflow=on  InputSameDT=on
  Out1 : Outport
  wires:
  In1/1 -> Product3/1
  In2/1 -> Product3/2
  Product3/1 -> Out1/1

== system gm_flightController/Flight Controller/ControlMixer/Product4 ==
  In1 : Inport
  In2 : Inport  Port=2
  Product4 : Sum  OutDataTypeStr=single  RndMeth=Zero  SampleTime=0.005  SaturateOnIntegerOverflow=on  InputSameDT=on
  Out1 : Outport
  wires:
  In1/1 -> Product4/1
  In2/1 -> Product4/2
  Product4/1 -> Out1/1

== system gm_flightController/Flight Controller/ControlMixer/Product5 ==
  In1 : Inport
  In2 : Inport  Port=2
  Product5 : Sum  OutDataTypeStr=single  RndMeth=Zero  SampleTime=0.005  SaturateOnIntegerOverflow=on  InputSameDT=on
  Out1 : Outport
  wires:
  In1/1 -> Product5/1
  In2/1 -> Product5/2
  Product5/1 -> Out1/1

== system gm_flightController/Flight Controller/ControlMixer/Product6 ==
  In1 : Inport
  In2 : Inport  Port=2
  Product6 : Sum  OutDataTypeStr=single  RndMeth=Zero  SampleTime=0.005  SaturateOnIntegerOverflow=on  InputSameDT=on
  Out1 : Outport
  wires:
  In1/1 -> Product6/1
  In2/1 -> Product6/2
  Product6/1 -> Out1/1

== system gm_flightController/Flight Controller/ControlMixer/Product7 ==
  In1 : Inport
  In2 : Inport  Port=2
  Product7 : Sum  OutDataTypeStr=single  RndMeth=Zero  SampleTime=0.005  SaturateOnIntegerOverflow=on  InputSameDT=on
  Out1 : Outport
  wires:
  In1/1 -> Product7/1
  In2/1 -> Product7/2
  Product7/1 -> Out1/1

== system gm_flightController/Flight Controller/ControlMixer/Product8 ==
  In1 : Inport
  In2 : Inport  Port=2
  Product8 : Sum  OutDataTypeStr=single  RndMeth=Zero  SampleTime=0.005  SaturateOnIntegerOverflow=on  InputSameDT=on
  Out1 : Outport
  wires:
  In1/1 -> Product8/1
  In2/1 -> Product8/2
  Product8/1 -> Out1/1

== system gm_flightController/Flight Controller/ControlMixer/Product9 ==
  In1 : Inport
  In2 : Inport  Port=2
  Product9 : Sum  OutDataTypeStr=single  RndMeth=Zero  SampleTime=0.005  SaturateOnIntegerOverflow=on  InputSameDT=on
  Out1 : Outport
  wires:
  In1/1 -> Product9/1
  In2/1 -> Product9/2
  Product9/1 -> Out1/1

== system gm_flightController/Flight Controller/ControlMixer/mul_Product_dotp_0 ==
  In1 : Inport
  In2 : Inport  Port=2
  mul_Product_dotp_0 : Product  Inputs=**  OutDataTypeStr=single  SampleTime=0.005  RndMeth=Zero
  Out1 : Outport
  wires:
  In1/1 -> mul_Product_dotp_0/1
  In2/1 -> mul_Product_dotp_0/2
  mul_Product_dotp_0/1 -> Out1/1

== system gm_flightController/Flight Controller/ControlMixer/mul_Product_dotp_01 ==
  In1 : Inport
  In2 : Inport  Port=2
  mul_Product_dotp_01 : Product  Inputs=**  OutDataTypeStr=single  SampleTime=0.005  RndMeth=Zero
  Out1 : Outport
  wires:
  In1/1 -> mul_Product_dotp_01/1
  In2/1 -> mul_Product_dotp_01/2
  mul_Product_dotp_01/1 -> Out1/1

== system gm_flightController/Flight Controller/ControlMixer/mul_Product_dotp_02 ==
  In1 : Inport
  In2 : Inport  Port=2
  mul_Product_dotp_02 : Product  Inputs=**  OutDataTypeStr=single  SampleTime=0.005  RndMeth=Zero
  Out1 : Outport
  wires:
  In1/1 -> mul_Product_dotp_02/1
  In2/1 -> mul_Product_dotp_02/2
  mul_Product_dotp_02/1 -> Out1/1

== system gm_flightController/Flight Controller/ControlMixer/mul_Product_dotp_03 ==
  In1 : Inport
  In2 : Inport  Port=2
  mul_Product_dotp_03 : Product  Inputs=**  OutDataTypeStr=single  SampleTime=0.005  RndMeth=Zero
  Out1 : Outport
  wires:
  In1/1 -> mul_Product_dotp_03/1
  In2/1 -> mul_Product_dotp_03/2
  mul_Product_dotp_03/1 -> Out1/1

== system gm_flightController/Flight Controller/ControlMixer/mul_Product_dotp_1 ==
  In1 : Inport
  In2 : Inport  Port=2
  mul_Product_dotp_1 : Product  Inputs=**  OutDataTypeStr=single  SampleTime=0.005  RndMeth=Zero
  Out1 : Outport
  wires:
  In1/1 -> mul_Product_dotp_1/1
  In2/1 -> mul_Product_dotp_1/2
  mul_Product_dotp_1/1 -> Out1/1

== system gm_flightController/Flight Controller/ControlMixer/mul_Product_dotp_11 ==
  In1 : Inport
  In2 : Inport  Port=2
  mul_Product_dotp_11 : Product  Inputs=**  OutDataTypeStr=single  SampleTime=0.005  RndMeth=Zero
  Out1 : Outport
  wires:
  In1/1 -> mul_Product_dotp_11/1
  In2/1 -> mul_Product_dotp_11/2
  mul_Product_dotp_11/1 -> Out1/1

== system gm_flightController/Flight Controller/ControlMixer/mul_Product_dotp_12 ==
  In1 : Inport
  In2 : Inport  Port=2
  mul_Product_dotp_12 : Product  Inputs=**  OutDataTypeStr=single  SampleTime=0.005  RndMeth=Zero
  Out1 : Outport
  wires:
  In1/1 -> mul_Product_dotp_12/1
  In2/1 -> mul_Product_dotp_12/2
  mul_Product_dotp_12/1 -> Out1/1

== system gm_flightController/Flight Controller/ControlMixer/mul_Product_dotp_13 ==
  In1 : Inport
  In2 : Inport  Port=2
  mul_Product_dotp_13 : Product  Inputs=**  OutDataTypeStr=single  SampleTime=0.005  RndMeth=Zero
  Out1 : Outport
  wires:
  In1/1 -> mul_Product_dotp_13/1
  In2/1 -> mul_Product_dotp_13/2
  mul_Product_dotp_13/1 -> Out1/1

== system gm_flightController/Flight Controller/ControlMixer/mul_Product_dotp_2 ==
  In1 : Inport
  In2 : Inport  Port=2
  mul_Product_dotp_2 : Product  Inputs=**  OutDataTypeStr=single  SampleTime=0.005  RndMeth=Zero
  Out1 : Outport
  wires:
  In1/1 -> mul_Product_dotp_2/1
  In2/1 -> mul_Product_dotp_2/2
  mul_Product_dotp_2/1 -> Out1/1

== system gm_flightController/Flight Controller/ControlMixer/mul_Product_dotp_21 ==
  In1 : Inport
  In2 : Inport  Port=2
  mul_Product_dotp_21 : Product  Inputs=**  OutDataTypeStr=single  SampleTime=0.005  RndMeth=Zero
  Out1 : Outport
  wires:
  In1/1 -> mul_Product_dotp_21/1
  In2/1 -> mul_Product_dotp_21/2
  mul_Product_dotp_21/1 -> Out1/1

== system gm_flightController/Flight Controller/ControlMixer/mul_Product_dotp_22 ==
  In1 : Inport
  In2 : Inport  Port=2
  mul_Product_dotp_22 : Product  Inputs=**  OutDataTypeStr=single  SampleTime=0.005  RndMeth=Zero
  Out1 : Outport
  wires:
  In1/1 -> mul_Product_dotp_22/1
  In2/1 -> mul_Product_dotp_22/2
  mul_Product_dotp_22/1 -> Out1/1

== system gm_flightController/Flight Controller/ControlMixer/mul_Product_dotp_23 ==
  In1 : Inport
  In2 : Inport  Port=2
  mul_Product_dotp_23 : Product  Inputs=**  OutDataTypeStr=single  SampleTime=0.005  RndMeth=Zero
  Out1 : Outport
  wires:
  In1/1 -> mul_Product_dotp_23/1
  In2/1 -> mul_Product_dotp_23/2
  mul_Product_dotp_23/1 -> Out1/1

== system gm_flightController/Flight Controller/ControlMixer/mul_Product_dotp_3 ==
  In1 : Inport
  In2 : Inport  Port=2
  mul_Product_dotp_3 : Product  Inputs=**  OutDataTypeStr=single  SampleTime=0.005  RndMeth=Zero
  Out1 : Outport
  wires:
  In1/1 -> mul_Product_dotp_3/1
  In2/1 -> mul_Product_dotp_3/2
  mul_Product_dotp_3/1 -> Out1/1

== system gm_flightController/Flight Controller/ControlMixer/mul_Product_dotp_31 ==
  In1 : Inport
  In2 : Inport  Port=2
  mul_Product_dotp_31 : Product  Inputs=**  OutDataTypeStr=single  SampleTime=0.005  RndMeth=Zero
  Out1 : Outport
  wires:
  In1/1 -> mul_Product_dotp_31/1
  In2/1 -> mul_Product_dotp_31/2
  mul_Product_dotp_31/1 -> Out1/1

== system gm_flightController/Flight Controller/ControlMixer/mul_Product_dotp_32 ==
  In1 : Inport
  In2 : Inport  Port=2
  mul_Product_dotp_32 : Product  Inputs=**  OutDataTypeStr=single  SampleTime=0.005  RndMeth=Zero
  Out1 : Outport
  wires:
  In1/1 -> mul_Product_dotp_32/1
  In2/1 -> mul_Product_dotp_32/2
  mul_Product_dotp_32/1 -> Out1/1

== system gm_flightController/Flight Controller/ControlMixer/mul_Product_dotp_33 ==
  In1 : Inport
  In2 : Inport  Port=2
  mul_Product_dotp_33 : Product  Inputs=**  OutDataTypeStr=single  SampleTime=0.005  RndMeth=Zero
  Out1 : Outport
  wires:
  In1/1 -> mul_Product_dotp_33/1
  In2/1 -> mul_Product_dotp_33/2
  mul_Product_dotp_33/1 -> Out1/1

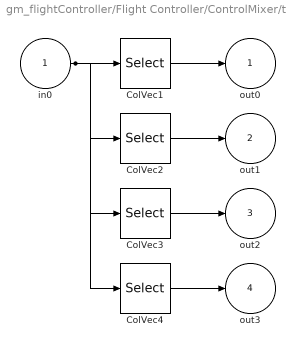
== system gm_flightController/Flight Controller/ControlMixer/t ==
  in0 : Inport
  ColVec1 : Selector  NumberOfDimensions=2  IndexOptions=Select all,Index vector (dialog)  Indices=1,1  OutputSizes=1,1
  ColVec2 : Selector  NumberOfDimensions=2  IndexOptions=Select all,Index vector (dialog)  Indices=1,2  OutputSizes=1,1
  ColVec3 : Selector  NumberOfDimensions=2  IndexOptions=Select all,Index vector (dialog)  Indices=1,3  OutputSizes=1,1
  ColVec4 : Selector  NumberOfDimensions=2  IndexOptions=Select all,Index vector (dialog)  Indices=1,4  OutputSizes=1,1
  out0 : Outport
  out1 : Outport  Port=2
  out2 : Outport  Port=3
  out3 : Outport  Port=4
  wires:
  in0/1 -> ColVec1/1, ColVec2/1, ColVec3/1, ColVec4/1
  ColVec1/1 -> out0/1
  ColVec2/1 -> out1/1
  ColVec3/1 -> out2/1
  ColVec4/1 -> out3/1

== system gm_flightController/Flight Controller/XY-to-reference-orientation/D_xy ==
  In1 : Inport
  In2 : Inport  Port=2
  D_xy : Product  Inputs=**  OutDataTypeStr=single  SampleTime=0.005  SaturateOnIntegerOverflow=on
  Out1 : Outport
  wires:
  In1/1 -> D_xy/1
  In2/1 -> D_xy/2
  D_xy/1 -> Out1/1

== system gm_flightController/Flight Controller/XY-to-reference-orientation/Gain_unaryminus ==
  In1 : Inport
  Gain_unaryminus : UnaryMinus  SampleTime=0.005
  Out1 : Outport
  wires:
  In1/1 -> Gain_unaryminus/1
  Gain_unaryminus/1 -> Out1/1

== system gm_flightController/Flight Controller/XY-to-reference-orientation/P_xy ==
  In1 : Inport
  In2 : Inport  Port=2
  P_xy : Product  Inputs=**  OutDataTypeStr=single  SampleTime=0.005  SaturateOnIntegerOverflow=on
  Out1 : Outport
  wires:
  In1/1 -> P_xy/1
  In2/1 -> P_xy/2
  P_xy/1 -> Out1/1

== system gm_flightController/Flight Controller/XY-to-reference-orientation/Product ==
  In1 : Inport
  In2 : Inport  Port=2
  Product : Sum  OutDataTypeStr=single  RndMeth=Zero  SampleTime=0.005  SaturateOnIntegerOverflow=on  InputSameDT=on
  Out1 : Outport
  wires:
  In1/1 -> Product/1
  In2/1 -> Product/2
  Product/1 -> Out1/1

== system gm_flightController/Flight Controller/XY-to-reference-orientation/Product1 ==
  In1 : Inport
  In2 : Inport  Port=2
  Product1 : Sum  OutDataTypeStr=single  RndMeth=Zero  SampleTime=0.005  SaturateOnIntegerOverflow=on  InputSameDT=on
  Out1 : Outport
  wires:
  In1/1 -> Product1/1
  In2/1 -> Product1/2
  Product1/1 -> Out1/1

== system gm_flightController/Flight Controller/XY-to-reference-orientation/Saturation_LowerRelop ==
  In1 : Inport
  In2 : Inport  Port=2
  Saturation_LowerRelop : RelationalOperator  Operator=>  OutDataTypeStr=boolean  SampleTime=0.005  RndMeth=Nearest
  Out1 : Outport
  wires:
  In1/1 -> Saturation_LowerRelop/1
  In2/1 -> Saturation_LowerRelop/2
  Saturation_LowerRelop/1 -> Out1/1

== system gm_flightController/Flight Controller/XY-to-reference-orientation/Saturation_UpperRelop ==
  In1 : Inport
  In2 : Inport  Port=2
  Saturation_UpperRelop : RelationalOperator  Operator=<  OutDataTypeStr=boolean  SampleTime=0.005  RndMeth=Nearest
  Out1 : Outport
  wires:
  In1/1 -> Saturation_UpperRelop/1
  In2/1 -> Saturation_UpperRelop/2
  Saturation_UpperRelop/1 -> Out1/1

== system gm_flightController/Flight Controller/XY-to-reference-orientation/Sum17 ==
  In1 : Inport
  In2 : Inport  Port=2
  Sum17 : Sum  Inputs=+-  OutDataTypeStr=single  SampleTime=0.005  SaturateOnIntegerOverflow=on  InputSameDT=on
  Out1 : Outport
  wires:
  In1/1 -> Sum17/1
  In2/1 -> Sum17/2
  Sum17/1 -> Out1/1

== system gm_flightController/Flight Controller/XY-to-reference-orientation/Sum18 ==
  In1 : Inport
  In2 : Inport  Port=2
  Sum18 : Sum  OutDataTypeStr=single  SampleTime=0.005  SaturateOnIntegerOverflow=on  InputSameDT=on
  Out1 : Outport
  wires:
  In1/1 -> Sum18/1
  In2/1 -> Sum18/2
  Sum18/1 -> Out1/1

== system gm_flightController/Flight Controller/XY-to-reference-orientation/Trigonometric Function ==
  In1 : Inport
  Trigonometric Function : Trigonometry  Operator=sincos  SampleTime=0.005
  Out1 : Outport
  Out2 : Outport  Port=2
  wires:
  In1/1 -> Trigonometric Function/1
  Trigonometric Function/1 -> Out1/1
  Trigonometric Function/2 -> Out2/1

== system gm_flightController/Flight Controller/XY-to-reference-orientation/mul_Product_dotp_0 ==
  In1 : Inport
  In2 : Inport  Port=2
  mul_Product_dotp_0 : Product  Inputs=**  OutDataTypeStr=single  SampleTime=0.005  RndMeth=Zero
  Out1 : Outport
  wires:
  In1/1 -> mul_Product_dotp_0/1
  In2/1 -> mul_Product_dotp_0/2
  mul_Product_dotp_0/1 -> Out1/1

== system gm_flightController/Flight Controller/XY-to-reference-orientation/mul_Product_dotp_01 ==
  In1 : Inport
  In2 : Inport  Port=2
  mul_Product_dotp_01 : Product  Inputs=**  OutDataTypeStr=single  SampleTime=0.005  RndMeth=Zero
  Out1 : Outport
  wires:
  In1/1 -> mul_Product_dotp_01/1
  In2/1 -> mul_Product_dotp_01/2
  mul_Product_dotp_01/1 -> Out1/1

== system gm_flightController/Flight Controller/XY-to-reference-orientation/mul_Product_dotp_1 ==
  In1 : Inport
  In2 : Inport  Port=2
  mul_Product_dotp_1 : Product  Inputs=**  OutDataTypeStr=single  SampleTime=0.005  RndMeth=Zero
  Out1 : Outport
  wires:
  In1/1 -> mul_Product_dotp_1/1
  In2/1 -> mul_Product_dotp_1/2
  mul_Product_dotp_1/1 -> Out1/1

== system gm_flightController/Flight Controller/XY-to-reference-orientation/mul_Product_dotp_11 ==
  In1 : Inport
  In2 : Inport  Port=2
  mul_Product_dotp_11 : Product  Inputs=**  OutDataTypeStr=single  SampleTime=0.005  RndMeth=Zero
  Out1 : Outport
  wires:
  In1/1 -> mul_Product_dotp_11/1
  In2/1 -> mul_Product_dotp_11/2
  mul_Product_dotp_11/1 -> Out1/1

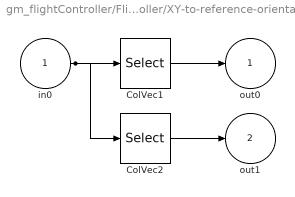
== system gm_flightController/Flight Controller/XY-to-reference-orientation/t ==
  in0 : Inport
  ColVec1 : Selector  NumberOfDimensions=2  IndexOptions=Select all,Index vector (dialog)  Indices=1,1  OutputSizes=1,1
  ColVec2 : Selector  NumberOfDimensions=2  IndexOptions=Select all,Index vector (dialog)  Indices=1,2  OutputSizes=1,1
  out0 : Outport
  out1 : Outport  Port=2
  wires:
  in0/1 -> ColVec1/1, ColVec2/1
  ColVec1/1 -> out0/1
  ColVec2/1 -> out1/1

== system gm_flightController/Flight Controller/Yaw/D_yaw ==
  In1 : Inport
  In2 : Inport  Port=2
  D_yaw : Product  Inputs=**  OutDataTypeStr=single  SampleTime=0.005
  Out1 : Outport
  wires:
  In1/1 -> D_yaw/1
  In2/1 -> D_yaw/2
  D_yaw/1 -> Out1/1

== system gm_flightController/Flight Controller/Yaw/P_yaw ==
  In1 : Inport
  In2 : Inport  Port=2
  P_yaw : Product  Inputs=**  OutDataTypeStr=single  SampleTime=0.005
  Out1 : Outport
  wires:
  In1/1 -> P_yaw/1
  In2/1 -> P_yaw/2
  P_yaw/1 -> Out1/1

== system gm_flightController/Flight Controller/Yaw/Sum1 ==
  In1 : Inport
  In2 : Inport  Port=2
  Sum1 : Sum  Inputs=+-  OutDataTypeStr=single  SampleTime=0.005  SaturateOnIntegerOverflow=on  InputSameDT=on
  Out1 : Outport
  wires:
  In1/1 -> Sum1/1
  In2/1 -> Sum1/2
  Sum1/1 -> Out1/1
